simulink model "DCtoThreePhaseACInverter"  (R2020a)
settings: Solver=VariableStepAuto  StartTime=0.0  StopTime=10.0  RelTol=1e-3
settings Model: Creator=Sony  LastModifiedBy=Sony

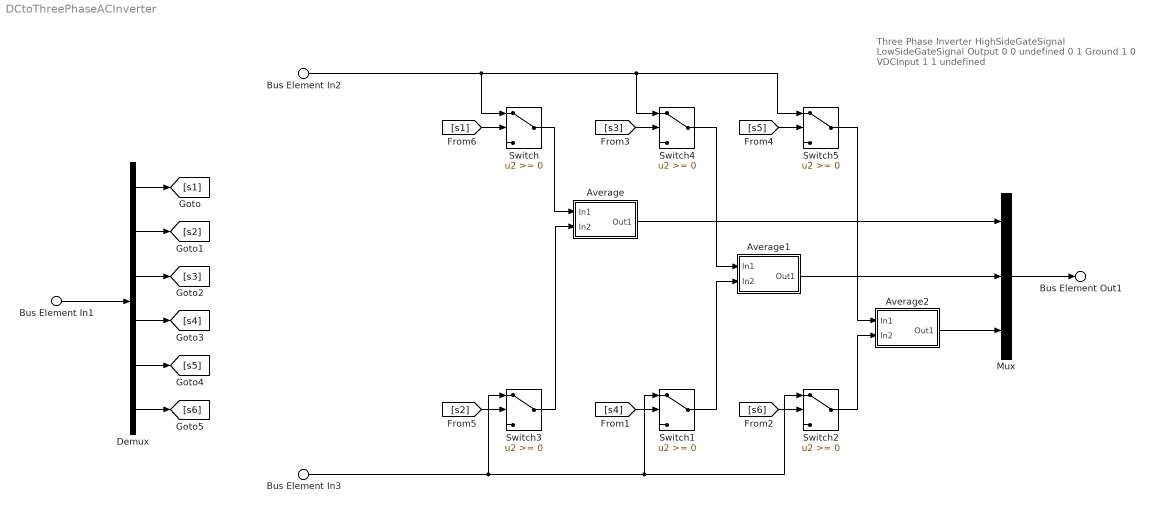
== system DCtoThreePhaseACInverter ==
  note: Three Phase Inverter
      | HighSideGateSignal LowSideGateSignal Output
      | 0 0 undefined
      | 0 1 Ground
      | 1 0 VDCInput
      | 1 1 undefined
  Bus Element In2 : Inport  PortName=DC Voltage VDC
  Bus Element In3 : Inport  Port=2  PortName=DC Ground
  Bus Element In1 : Inport  Port=3  PortName=Gatings
  Average : Subsystem
  Average1 : Subsystem
  Average2 : Subsystem
  Demux : Demux  Outputs=6
  Mux : Mux  Inputs=3
  Switch{,1..5} (6 alike) : Switch
  Bus Element Out1 : Outport  PortName=AC Stator Voltages VABC
  wires:
  Switch4/1 -> Average1/1(In1)
  Switch5/1 -> Average2/1(In1)
  [s6] -> Switch2/2
  [s5] -> Switch5/2
  [s4] -> Switch1/2
  Bus Element In1/1 -> Demux/1
  Average1/1(Out1) -> Mux/2
  Switch1/1 -> Average1/2(In2)
  [s3] -> Switch4/2
  [s2] -> Switch3/2
  Demux/4 -> [s4]
  Switch3/1 -> Average/2(In2)
  Switch2/1 -> Average2/2(In2)
  Demux/1 -> [s1]
  Switch/1 -> Average/1(In1)
  Average/1(Out1) -> Mux/1
  Bus Element In3/1 -> Switch3/1, Switch2/1, Switch1/1
  Demux/2 -> [s2]
  Demux/5 -> [s5]
  Demux/3 -> [s3]
  Demux/6 -> [s6]
  Average2/1(Out1) -> Mux/3
  [s1] -> Switch/2
  Bus Element In2/1 -> Switch/1, Switch5/1, Switch4/1
  Mux/1 -> Bus Element Out1/1

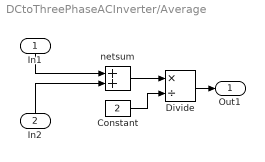
== system DCtoThreePhaseACInverter/Average ==
  In1 : Inport
  In2 : Inport  Port=2
  Constant : Constant  Value=2
  Divide : Product  Inputs=*/
  netsum : Sum  Inputs=2  InputSameDT=on  SaturateOnIntegerOverflow=on  OutDataTypeStr=Inherit: Same as first input
  Out1 : Outport
  wires:
  In1/1 -> netsum/1
  Constant/1 -> Divide/2
  Divide/1 -> Out1/1
  In2/1 -> netsum/2
  netsum/1 -> Divide/1

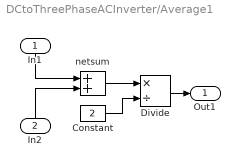
== system DCtoThreePhaseACInverter/Average1 ==
  In1 : Inport
  In2 : Inport  Port=2
  Constant : Constant  Value=2
  Divide : Product  Inputs=*/
  netsum : Sum  Inputs=2  InputSameDT=on  SaturateOnIntegerOverflow=on  OutDataTypeStr=Inherit: Same as first input
  Out1 : Outport
  wires:
  In1/1 -> netsum/1
  Constant/1 -> Divide/2
  Divide/1 -> Out1/1
  In2/1 -> netsum/2
  netsum/1 -> Divide/1

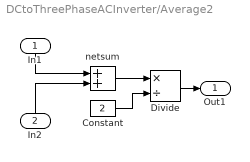
== system DCtoThreePhaseACInverter/Average2 ==
  In1 : Inport
  In2 : Inport  Port=2
  Constant : Constant  Value=2
  Divide : Product  Inputs=*/
  netsum : Sum  Inputs=2  InputSameDT=on  SaturateOnIntegerOverflow=on  OutDataTypeStr=Inherit: Same as first input
  Out1 : Outport
  wires:
  In1/1 -> netsum/1
  Constant/1 -> Divide/2
  Divide/1 -> Out1/1
  In2/1 -> netsum/2
  netsum/1 -> Divide/1
